simulink model "speedgoat_IO316_CI_01547"  (R2017a)
settings: Solver=FixedStepDiscrete  StartTime=0.0  StopTime=inf  RelTol=1e-3  EnableMultiTasking=on
PreLoadFcn:
  | if ~exist('Ts', 'var')
  | Ts = 0.001;
  | end
  | if ~exist('FPGA_Frequency', 'var')
  | FPGA_Frequency = 75000000;
  | end
libraries: slrtlib x4, simulink x4, speedgoatlib_fpga x3, speedgoatlib_fpga_spi x2
settings Model: SimulationMode=external  Creator=bvongunten  LastModifiedBy=mc-user
settings SolverCC: EnableConcurrentExecution=on
settings DataIOCC: SaveFormat=StructureWithTime
settings OptimizationCC: BlockReduction=off  OptimizeBlockIOStorage=off  BufferReuse=off  GlobalBufferReuse=off  ExpressionFolding=off  LocalBlockOutputs=off  LifeSpan=inf
settings DebuggingCC: UnderspecifiedInitializationDetection=Classic  MergeDetectMultiDrivingBlocksExec=none  UnconnectedInputMsg=none  UnconnectedOutputMsg=none  UnconnectedLineMsg=none  SFExecutionAtInitializationDiag=none
settings HardwareCC: ProdBitPerPointer=32  ProdBitPerSizeT=32  ProdBitPerPtrDiffT=32  ProdLargestAtomicFloat=None  ProdWordSize=32  ProdLongLongMode=on  ProdHWDeviceType=Generic->32-bit x86 compatible
settings ModelReferenceCC: PropagateSignalLabelsOutOfModel=off
settings RTWCC: SystemTargetFile=slrt.tlc  TemplateMakefile=slrt_default_tmf  Description=Simulink Real-Time  RTWCompilerOptimization=on
settings SimulinkRealTimeCC: RL32LogTETModifier=off

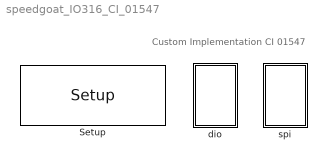
== system speedgoat_IO316_CI_01547 ==
  note: Custom Implementation CI 01547
  Setup : speedgoatlib_fpga/Setup/Setup  board=IO316  id=1  frontIO=None  rearIO=None  bitstreamFile=speedgoat_IO316_CI_01547  ProgSpiFlash=off  ProgBPIFlash=off  pciSlot=-1  PullRPort0=pull-up 3.3V  VioPort0=3.3V  PullRPort1=pull-up 3.3V  VioPort1=3.3V  PullRPort2=pull-up 3.3V  VioPort2=3.3V  PullRPort3=pull-up 3.3V  VioPort3=3.3V  PullRPort4=pull-up 3.3V  VioPort4=3.3V  PullRPort5=pull-up 3.3V  VioPort5=3.3V  PullRPort6=pull-up 3.3V  VioPort6=3.3V  PullRPort15=pull-up 3.3V  PullRPort31=pull-up 3.3V  PullRPort47=pull-up 3.3V  PullRPort63=pull-up 3.3V
      settings: SourceProductName=Simulink Real-Time: Speedgoat I/O Driver Library
  dio : Subsystem
  spi : Subsystem

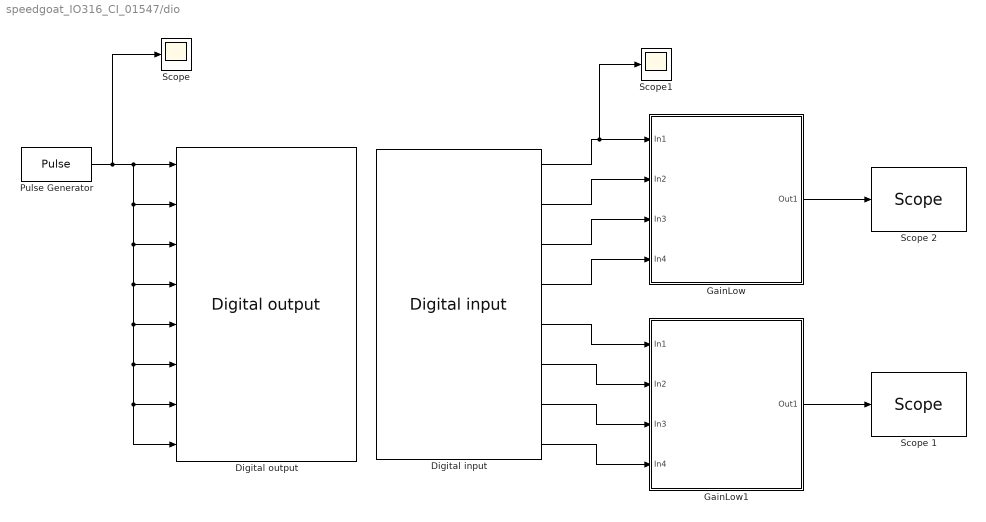
== system speedgoat_IO316_CI_01547/dio ==
  Digital input : speedgoatlib_fpga/Digital IO/Digital input  id=1  chan=[9:12, 25:28]  vectorizeOutput=off  ts=Ts  pciSlot=-1  board=IO316
      settings: SourceProductName=Simulink Real-Time: Speedgoat I/O Driver Library
  Digital output : speedgoatlib_fpga/Digital IO/Digital output  id=1  chan=[1:4,20:23]  init=[0]  reset=[0]  vectorizeInput=off  ts=Ts  pciSlot=-1  board=IO316
      settings: SourceProductName=Simulink Real-Time: Speedgoat I/O Driver Library
  GainLow : Subsystem
  GainLow1 : Subsystem
  Pulse Generator : DiscretePulseGenerator  Period=20  PulseWidth=10  SampleTime=Ts
  Scope : Scope
  Scope 1 : slrtlib/Displays and Logging/Scope   scopeno=1  scopetype=Target  autostart=on  viewmode=Graphical redraw  formatstr='%15.6f'  grid=on  ylimits=[0,0]  nosamples=250  noprepostsamples=0  interleave=1  triggermode=FreeRun  triggersignal=1  trigsignalfromport=off  triggerlevel=0.0  triggerslope=Either  triggerscope=1  triggersample=0  filename=data.dat  mode=Lazy  writesize=512  autorestart=off  dynamicfilemode=off  maxwritefilesize=512*1024^2
  Scope 2 : slrtlib/Displays and Logging/Scope   scopeno=2  scopetype=Target  autostart=on  viewmode=Graphical redraw  formatstr='%15.6f'  grid=on  ylimits=[0,0]  nosamples=250  noprepostsamples=0  interleave=1  triggermode=FreeRun  triggersignal=1  trigsignalfromport=off  triggerlevel=0.0  triggerslope=Either  triggerscope=1  triggersample=0  filename=data.dat  mode=Lazy  writesize=512  autorestart=off  dynamicfilemode=off  maxwritefilesize=512*1024^2
  Scope1 : Scope
  wires:
  Digital input/8 -> GainLow1/4(In4)
  Digital input/7 -> GainLow1/3(In3)
  Digital input/6 -> GainLow1/2(In2)
  Digital input/5 -> GainLow1/1(In1)
  GainLow1/1(Out1) -> Scope 1/1
  GainLow/1(Out1) -> Scope 2/1
  Digital input/4 -> GainLow/4(In4)
  Digital input/3 -> GainLow/3(In3)
  Digital input/2 -> GainLow/2(In2)
  Digital input/1 -> Scope1/1, GainLow/1(In1)
  Pulse Generator/1 -> Scope/1, Digital output/3, Digital output/4, Digital output/5, Digital output/6, Digital output/7, Digital output/8, Digital output/2, Digital output/1

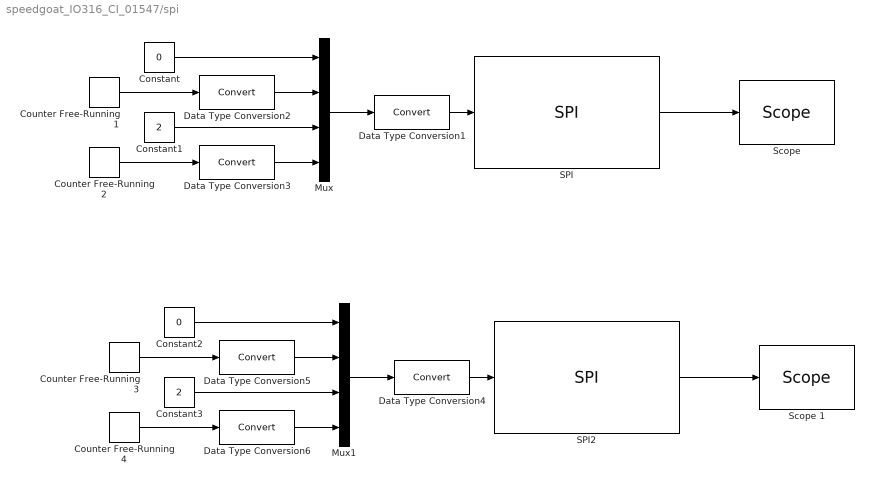
== system speedgoat_IO316_CI_01547/spi ==
  Constant : Constant  Value=0
  Constant1 : Constant  Value=2
  Constant2 : Constant  Value=0
  Constant3 : Constant  Value=2
  Counter Free-Running{1..4} (4 alike) : simulink/Sources/Counter Free-Running  NumBits=8  tsamp=-1
  Data Type Conversion{1..6} (6 alike) : DataTypeConversion
  Mux : Mux
  Mux1 : Mux
  SPI : speedgoatlib_fpga_spi/SPI  id=1  chan=[1]  ts=Ts  pciSlot=-1  board=IO316  cpol=[1]  cpha=[1]  masterNSlave=Master role  clockDivider=[40]  startDelay=[5]  interwordDelay=[0]  stopDelay=[5]  wordSize=[8]  frameSize=[4]  compensation=0  showTX=on  showRX=on  showCount=on
      settings: SourceProductName=Simulink Real-Time: Speedgoat I/O Driver Library
  SPI2 : speedgoatlib_fpga_spi/SPI  id=1  chan=[2]  ts=Ts  pciSlot=-1  board=IO316  cpol=[1]  cpha=[1]  masterNSlave=Slave role  clockDivider=[40]  startDelay=[5]  interwordDelay=[0]  stopDelay=[5]  wordSize=[8]  frameSize=[4]  compensation=0  showTX=on  showRX=on  showCount=on
      settings: SourceProductName=Simulink Real-Time: Speedgoat I/O Driver Library
  "Scope " : slrtlib/Displays and Logging/Scope   scopeno=3  scopetype=Target  autostart=on  viewmode=Numerical  formatstr='%15.6f'  grid=on  ylimits=[0,0]  nosamples=3  noprepostsamples=0  interleave=1  triggermode=FreeRun  triggersignal=1  trigsignalfromport=off  triggerlevel=0.0  triggerslope=Either  triggerscope=1  triggersample=0  filename=data.dat  mode=Lazy  writesize=512  autorestart=off  dynamicfilemode=off  maxwritefilesize=512*1024^2
  Scope 1 : slrtlib/Displays and Logging/Scope   scopeno=4  scopetype=Target  autostart=on  viewmode=Numerical  formatstr='%15.6f'  grid=on  ylimits=[0,0]  nosamples=3  noprepostsamples=0  interleave=1  triggermode=FreeRun  triggersignal=1  trigsignalfromport=off  triggerlevel=0.0  triggerslope=Either  triggerscope=1  triggersample=0  filename=data.dat  mode=Lazy  writesize=512  autorestart=off  dynamicfilemode=off  maxwritefilesize=512*1024^2
  wires:
  Data Type Conversion1/1 -> SPI/1
  Data Type Conversion3/1 -> Mux/4
  Counter Free-Running2/1 -> Data Type Conversion3/1
  Constant1/1 -> Mux/3
  Data Type Conversion2/1 -> Mux/2
  Mux/1 -> Data Type Conversion1/1
  Counter Free-Running1/1 -> Data Type Conversion2/1
  Constant/1 -> Mux/1
  SPI/1 -> "Scope "/1
  Data Type Conversion4/1 -> SPI2/1
  Data Type Conversion6/1 -> Mux1/4
  Counter Free-Running4/1 -> Data Type Conversion6/1
  Constant3/1 -> Mux1/3
  Data Type Conversion5/1 -> Mux1/2
  Mux1/1 -> Data Type Conversion4/1
  Counter Free-Running3/1 -> Data Type Conversion5/1
  Constant2/1 -> Mux1/1
  SPI2/1 -> Scope 1/1

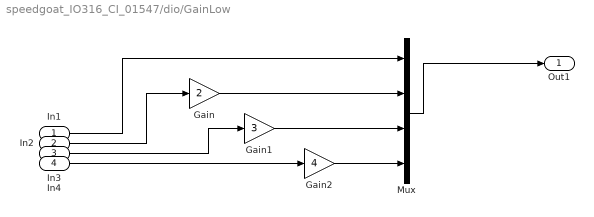
== system speedgoat_IO316_CI_01547/dio/GainLow ==
  In1 : Inport
  In2 : Inport  Port=2
  In3 : Inport  Port=3
  In4 : Inport  Port=4
  Gain : Gain  Gain=2
  Gain1 : Gain  Gain=3
  Gain2 : Gain  Gain=4
  Mux : Mux
  Out1 : Outport
  wires:
  In2/1 -> Gain/1
  In1/1 -> Mux/1
  In3/1 -> Gain1/1
  In4/1 -> Gain2/1
  Mux/1 -> Out1/1
  Gain/1 -> Mux/2
  Gain1/1 -> Mux/3
  Gain2/1 -> Mux/4

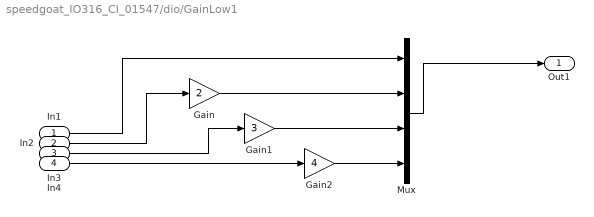
== system speedgoat_IO316_CI_01547/dio/GainLow1 ==
  In1 : Inport
  In2 : Inport  Port=2
  In3 : Inport  Port=3
  In4 : Inport  Port=4
  Gain : Gain  Gain=2
  Gain1 : Gain  Gain=3
  Gain2 : Gain  Gain=4
  Mux : Mux
  Out1 : Outport
  wires:
  In2/1 -> Gain/1
  In1/1 -> Mux/1
  In3/1 -> Gain1/1
  In4/1 -> Gain2/1
  Mux/1 -> Out1/1
  Gain/1 -> Mux/2
  Gain1/1 -> Mux/3
  Gain2/1 -> Mux/4
